simulink model "cepzn51"  (R2021a)
settings: Solver=VariableStepAuto  StartTime=0.0  StopTime=20000  RelTol=1e-3
values from neighbouring files (symbols this model uses):
  Ts = 0.5    [Distillation_Column_model_identification.m]    (also in Distillation_Column_model_variance.m; fourvary.m = 8)
libraries: dspsrcs4 x1
settings Model: Creator=dell  LastModifiedBy=dell

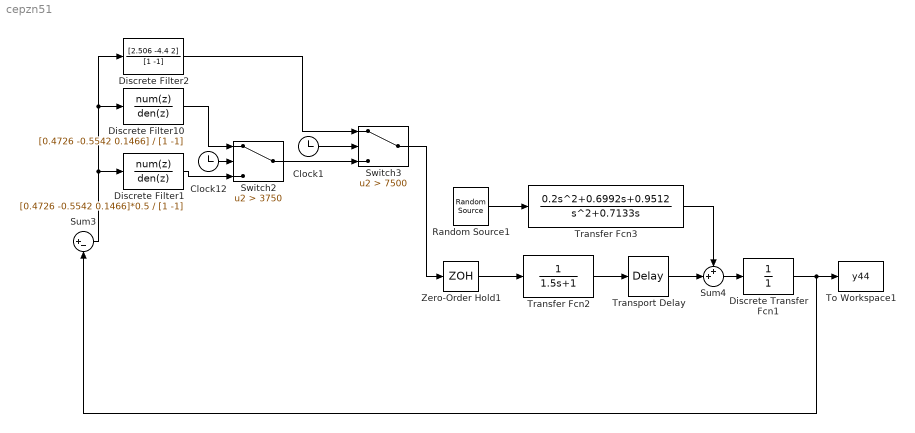
== system cepzn51 ==
  Clock1 : Clock
  Clock12 : Clock
  Discrete Transfer Fcn1 : DiscreteTransferFcn  Denominator=[1]  SampleTime=Ts
      mask Display: disp('sampler')
  Discrete Filter1 : DiscreteFilter  Numerator=[0.4726 -0.5542 0.1466]*0.5  Denominator=[1 -1]  SampleTime=Ts
  Discrete Filter10 : DiscreteFilter  Numerator=[0.4726 -0.5542 0.1466]  Denominator=[1 -1]  SampleTime=Ts
  Discrete Filter2 : DiscreteFilter  Numerator=[2.506 -4.4 2]  Denominator=[1 -1]  SampleTime=Ts
  Random Source1 : dspsrcs4/Random Source  SrcType=Gaussian  NormMethod=Ziggurat  CltLength=12  MinVal=-1  MaxVal=1  MeanVal=0  VarVal=1  RepMode=Specify seed  rawSeed=1  IsInherit=off  SampMode=Continuous  SampTime=1  SampFrame=1  DataType=Double  OutComplex=Real  OutputFrames=off
  Sum3 : Sum  Inputs=|+-
  Sum4 : Sum  Inputs=++|
  Switch2 : Switch  Criteria=u2 > Threshold  Threshold=3750
  Switch3 : Switch  Criteria=u2 > Threshold  Threshold=7500
  To Workspace1 : ToWorkspace  VariableName=y44  SampleTime=Ts
  Transfer Fcn2 : TransferFcn  Denominator=[1.5 1]
  Transfer Fcn3 : TransferFcn  Numerator=[0.2 0.6992 0.9512]  Denominator=[1 0.7133 0]
  Transport Delay : TransportDelay  DelayTime=5
  Zero-Order Hold1 : ZeroOrderHold  SampleTime=Ts
  wires:
  Discrete Transfer Fcn1/1 -> To Workspace1/1, Sum3/2
  Transport Delay/1 -> Sum4/2
  Transfer Fcn3/1 -> Sum4/1
  Random Source1/1 -> Transfer Fcn3/1
  Sum4/1 -> Discrete Transfer Fcn1/1
  Zero-Order Hold1/1 -> Transfer Fcn2/1
  Transfer Fcn2/1 -> Transport Delay/1
  Sum3/1 -> Discrete Filter1/1, Discrete Filter10/1, Discrete Filter2/1
  Discrete Filter10/1 -> Switch2/1
  Switch2/1 -> Switch3/3
  Discrete Filter2/1 -> Switch3/1
  Switch3/1 -> Zero-Order Hold1/1
  Clock12/1 -> Switch2/2
  Discrete Filter1/1 -> Switch2/3
  Clock1/1 -> Switch3/2
